simulink model "run_quadrotor_2020a"  (R2020a)
settings: Solver=ode23  StartTime=0.0  StopTime=60  FixedStep=10/1000  MaxStep=0.01  MinStep=1/1000  RelTol=1e-5  EnableMultiTasking=on
InitFcn:
  | addpath('display/')
  | addpath('parameters/')
  | addpath('quadrotor_model')
  | addpath('tools/')
  | addpath('libs/RealTima_Pacer')
  | aerosonde_parameters
  | simulation_parameters
model workspace (MAT data in the model file):
  D1_podbor1 = 902.0676
  D1_podbor_psi = 334.133298018
  D1_podbor_y = 97.9069
  D_podbor_x = 10
  D_podbor_z = 10
  I1_podbor1 = 320.9285
  I1_podbor_psi = 2.71828630961
  I1_podbor_y = 0.6752
  I_podbor_x = 50
  I_podbor_z = 50
  P1_podbor1 = 7509.4
  P1_podbor_psi = 848.547345881
  P1_podbor_y = 264.9363
  P_podbor_x = 50
  P_podbor_z = 50
  theta_1_P_param : Simulink.Parameter (value not decoded)
  theta_1_P_paramCopy : Simulink.Parameter (value not decoded)
undefined symbols (not defined in the file or in its folder): drawQuadrotor, filter_freq, ln, MAV, plotmavstatevariables, setup_pid
libraries: simulink x11, checkpacklib x5, dspsigattribs x2, realtime_pacer_lib x1
(part 2 of 2)

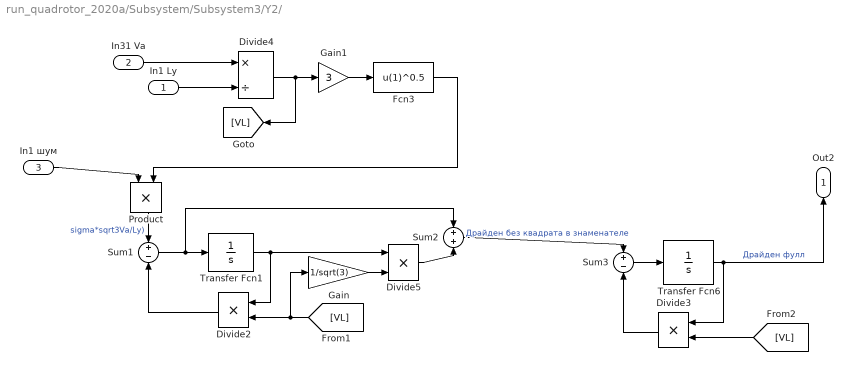
== system run_quadrotor_2020a/Subsystem/Subsystem3/Y2/  ==
  In1 Ly : Inport
  In31 Va : Inport  Port=2
  "In1 шум " : Inport  Port=3
  Divide2 : Product  Inputs=**
  Divide3 : Product  Inputs=**
  Divide4 : Product  Inputs=*/
  Divide5 : Product  Inputs=**
  Fcn3 : Fcn  Expr=u(1)^0.5
  Gain : Gain  Gain=1/sqrt(3)
  Gain1 : Gain  Gain=3
  Product : Product
  Sum1 : Sum  Inputs=+-
  Sum2 : Sum
  Sum3 : Sum  Inputs=+-
  Transfer Fcn1 : TransferFcn  Denominator="[1  0]"
  Transfer Fcn6 : TransferFcn  Denominator="[1  0]"
  Out2 : Outport
  wires:
  Divide4/1 -> [VL], Gain1/1
  Sum1/1 -> Transfer Fcn1/1, Sum2/1
  Sum2/1 -> Sum3/1  "Драйден без квадрата в знаменателе"
  Transfer Fcn1/1 -> Divide2/1, Divide5/1
  Divide2/1 -> Sum1/2
  Gain1/1 -> Fcn3/1
  In31 Va/1 -> Divide4/1
  In1 Ly/1 -> Divide4/2
  [VL] -> Gain/1, Divide2/2
  Gain/1 -> Divide5/2
  Divide5/1 -> Sum2/2
  Transfer Fcn6/1 -> Out2/1, Divide3/1  "Драйден фулл"
  Divide3/1 -> Sum3/2
  Sum3/1 -> Transfer Fcn6/1
  [VL] -> Divide3/2
  "In1 шум "/1 -> Product/1
  Fcn3/1 -> Product/2
  Product/1 -> Sum1/1  "sigma*sqrt3Va/Ly)"

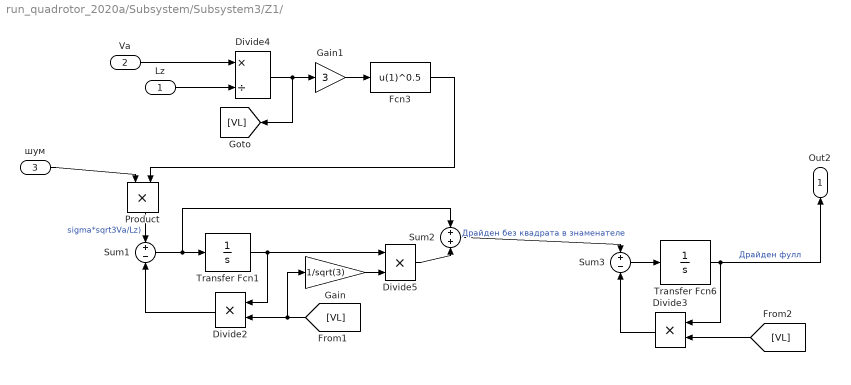
== system run_quadrotor_2020a/Subsystem/Subsystem3/Z1/  ==
  Lz : Inport
  Va : Inport  Port=2
  "шум " : Inport  Port=3
  Divide2 : Product  Inputs=**
  Divide3 : Product  Inputs=**
  Divide4 : Product  Inputs=*/
  Divide5 : Product  Inputs=**
  Fcn3 : Fcn  Expr=u(1)^0.5
  Gain : Gain  Gain=1/sqrt(3)
  Gain1 : Gain  Gain=3
  Product : Product
  Sum1 : Sum  Inputs=+-
  Sum2 : Sum
  Sum3 : Sum  Inputs=+-
  Transfer Fcn1 : TransferFcn  Denominator="[1  0]"
  Transfer Fcn6 : TransferFcn  Denominator="[1  0]"
  Out2 : Outport
  wires:
  Divide4/1 -> [VL], Gain1/1
  Sum1/1 -> Transfer Fcn1/1, Sum2/1
  Sum2/1 -> Sum3/1  "Драйден без квадрата в знаменателе"
  Transfer Fcn1/1 -> Divide2/1, Divide5/1
  Divide2/1 -> Sum1/2
  Gain1/1 -> Fcn3/1
  Va/1 -> Divide4/1
  Lz/1 -> Divide4/2
  [VL] -> Gain/1, Divide2/2
  Gain/1 -> Divide5/2
  Divide5/1 -> Sum2/2
  Transfer Fcn6/1 -> Out2/1, Divide3/1  "Драйден фулл"
  Divide3/1 -> Sum3/2
  Sum3/1 -> Transfer Fcn6/1
  [VL] -> Divide3/2
  "шум "/1 -> Product/1
  Fcn3/1 -> Product/2
  Product/1 -> Sum1/1  "sigma*sqrt3Va/Lz)"

== matlab function run_quadrotor_2020a/Subsystem1/In what the force, bro? ==
  data: Vb input; Fb output; Wb input
function Fb = AerialDrag(Vb, Wb)
    rho = 1.19;
    Va_vec = Vb - Wb;  % w - wind, v - ground speed; body frame
    Va = norm(Va_vec);
    alpha = atan2(Va_vec(2), Va_vec(1));    % attack angle
    beta = atan2(Va_vec(3), Va_vec(1));     % скольжения angle
    
    Va_0 = 10; % скорость, для которой рассчитаны зависимости сил
    rho_0 = 1.225;  % плотность воздуха при выведении зависимостей сил
%     C_0 = 0.715 / (0.5*rho_0*Va_0^2);  % if alpha = 0, beta = 0;
    % ----------------------------------------------------
    % alpha angle
    alpha = abs(alpha);
    alpha = sign(alpha)*mod(alpha, 180);
    alpha = alpha + 180 * sign(90-alpha)*(abs(alpha)>90);
    if alpha >= 0 && alpha <= 20
        F_xy = 0.6969 + 0.0022*(alpha+2.3409).^2;
    elseif alpha > 20 && alpha <= 90
        F_xy = -0.000435*alpha^2 + 0.098161*alpha - 0.007685;
%         C_d = 5.5300 - 4.3500e-04*(alpha - 112.8287)^2;
    elseif alpha >= -20 && alpha < 0
        F_xy = 0.6969 + 0.0022*(-alpha+2.3409).^2;
    else
        F_xy = 5.5300 - 4.3500e-04*(-alpha - 112.8287)^2;
    end
%     C_D_alpha = F_0 / (0.5*rho_0*Va_0^2) - C_0;
%     C_D_alpha = F_0 / (0.5*rho_0*Va_0^2);
        C_xy = F_xy / (0.5*rho_0*Va_0^2);
        C_x = C_xy * cos(alpha);
        C_y = C_xy * sin(alpha);
        
        
    
    %-----------------------------------------------------
    % beta angle
    b = abs(beta);
    b = sign(b)*mod(b, 180);
    b = b + 180 * sign(90-b)*(abs(b)>90);
    if b >= 0 && b <= 10
        F_xz = 2.81659e-7*b^6 - 5.42002e-6*b^5 + 0.0000194033*b^4 + 0.000149284*b^3 - 0.000766659*b^2 + 0.00100311*b + 0.715;
    elseif b > 10 && b <= 32
        F_xz = 0.000072941364*b^2+0.004725990899*b+0.676768850038;
    elseif b > 32 && b <= 47
        F_xz = 0.000014983590*b^3-0.002016505717*b^2+0.091338487517*b-0.446303186240;
    elseif b > 47 && b <= 66
        F_xz = -0.000005286789*b^3+0.000705178007*b^2-0.030877630605*b+1.390205322532;
    elseif b > 66 && b <= 90
        F_xz = 0.000000379469*b^3+0.000021666922*b^2-0.013615025702*b+1.599215019960;            
    else
        F_xz = 0;
    end
    C_xz = F_xz / (0.5*rho_0*Va_0^2);
    C_z = C_xz * sin(beta);
%     C_D_beta = F0 / (0.5*rho_0*Va_0^2) - C_0;
    
    
    % ----------------------------------------------
    % Drug force
%     F_D = 0.5*rho*Va^2 * (C_0 + alpha*C_D_alpha + beta*C_D_beta);
    
%     F_D = 0.5*rho*Va^2 * (C_D_alpha);
%     
%     Fa = [
%         (-1)*F_D;
%         0;
%         0;
%     ];  % в скоростной СК
%     c_a = cos(alpha); s_a = sin(alpha);
%     c_b = cos(beta); s_b = sin(beta);
%     % TODO: перепроверить, кто в кого переводитъ
%     R_a_b = [c_a*c_b -s_a*c_b s_b; s_a c_a 0; -c_a*s_b s_a*s_b c_b];    % из скоростной с связанную
% %     R_b_a = [ c_a s_a 0; -s_a c_a 0; 0 0 1];    % из связанной в скоростную
% %     Fb = R_b_a' * Fa;
%         Fb = R_a_b * Fa;
    Fb = (-1)*(1/2)*rho*Va^2 * [C_x; C_y; C_z];
end

== matlab function run_quadrotor_2020a/Motor Controller1 ==
  data: N output; u input
% Calculate desired motor speeds N with given control u
function N = fcn(u)
u_T = u(1);
u_x = u(2);
u_y = u(3);
u_z = u(4);

% NN = 0.25*[u_T+u_z u_T+u_z u_T-u_z u_T-u_z]';
% A = (1/4)*[
%     1 1;
%     1 1;
%     1 -1;
%     1 -1
% ];
A = (1/4)*[
    1 1 1 1;
    1 -1 -1 1;
    1 -1 1 -1;
    1 1 -1 -1;
];

NN = A*[u_T; u_x; u_y; u_z];
NN = max(NN, 0);
N = sqrt(NN);

% If we want at once disarm motors (landing etc.)
% if disable_motors == 7
%     N = zeros(4,1);
% end

== matlab function run_quadrotor_2020a/REG1/Flush integrators commandor/MATLAB Function ==
  data: mode_vec input; prev_mode_vec input; command output; prev_command input; mode_vec output
function [command, mode_vec]  = fcn(mode_vec, prev_mode_vec, prev_command)
    command = prev_command;
%     persistent prev_mode;
%     if isempty(prev_mode)
%        prev_mode = -1; 
%     end
    if prev_mode_vec == mode_vec
        return
    end
%     prev_mode = mode;
    % command: [ theta x y]
    
    mode = FlightMode(mode_vec);
    prev_mode = FlightMode(prev_mode_vec);
    phi = 1; x = 2; y = 3;
    
    % если изменился канал х
    if mode.get('x') ~= prev_mode.get('x')
        command(x) = double(~prev_command(x));
        if mode.get('x') == 0 || mode.get('x') == 1
            command(phi) = double(~prev_command(phi));
        end
    end
    
    if mode.get('y') ~= prev_mode.get('y')
        command(y) = double(~prev_command(y));
    end
    
    

%     if mode == 2 || mode == 0
%         command = double(~prev_command);
%     end
%     if mode == 3 || mode == 5
%         command(2) = double(~prev_command(2));
%     end
%     if mode == 4 || mode == 5 || mode == 6
%         command(3) = double(~prev_command(3));
%     end

== matlab function run_quadrotor_2020a/Subsystem/Subsystem3/MATLAB Function1 ==
  data: euler input; Wb output; va input
function Wb = rotate_g_b(euler, va)
R = getRotationMatrix(euler);
vay=0; vaz=0;
Va = [-va; vay; vaz];
Wb = R*Va;

function R = getRotationMatrix(angles)
    phi = 1; t = 2; psi = 3; %indices
    s = sin(angles);
    c = cos(angles);
    R = [
        c(t)*c(psi) s(t)    -c(t)*s(psi);
        -c(phi)*s(t)*c(psi)+s(phi)*s(psi) c(phi)*c(t) c(phi)*s(t)*s(psi)+s(phi)*c(psi);
        s(phi)*s(t)*c(psi)+c(phi)*s(psi)  -s(phi)*c(t)    -s(psi)*s(t)*s(phi)+c(psi)*c(phi);
    ];

== matlab function run_quadrotor_2020a/Subsystem1/Old Force ==
  data: v input; F output; w input
function F = AerialDrag(v, w)
    rho = 1.19;
    S = [5573 59852 6884] / (100*10)^2;
    C = 1.0;
    Va = v - w;  % w - wind, v - ground speed;
    % S - характерная площадь
    F = - C * rho * Va.^2/2 .* S';
end

== matlab function run_quadrotor_2020a/REG1/g -> g_1(psi) ==
  data: g_vec input; g1_vec output; psi input
% Поворот вектора глобальной СК в полусвязанную на угол рыскания
function g1_vec = fcn(g_vec, psi)

c_p = cos(psi); s_p = sin(psi);
R = [c_p 0 -s_p; 0 1 0; s_p 0 c_p];
g1_vec = R * g_vec;

== matlab function run_quadrotor_2020a/Sensors Real/MATLAB Function ==
  data: v input; d_v input; ang input; a_prop output; w input
% Считает проекции кажущегося ускорения,
% эмуляция показателей акселерометра
% @v - скорость в связанной СК
% @d_v - производная скорости выше
% @ang - углы Эйлера
% @w - угловая скорость в проекциях на связанные оси
function a_prop = fcn(v, d_v, ang, w)
phi = ang(1);
theta = ang(2); 
g = 9.81;

% coriolis = [
%     w(3)*v(2) - w(2)*v(3);
%     w(1)*v(3) - w(3)*v(1);
%     w(2)*v(1) - w(1)*v(2)
% ];

coriolis = cross(v, w);

R = [
    sin(theta);
    cos(phi)*cos(theta);
    -sin(phi)*cos(theta)
];

a_prop = d_v - coriolis + R*g;

% a_prop(1) = d_v(1) - (w(3)*v(2) - w(2)*v(3)) + g*sin(theta);
% a_prop(2) = d_v(2) - (w(1)*v(3) - w(3)*v(1)) + g*cos(phi)*cos(theta);
% a_prop(3) = d_v(3) - (w(2)*v(1) - w(1)*v(2)) - g*sin(phi)*cos(theta);

== matlab function run_quadrotor_2020a/desired fixed1 ==
  data: des_state output; MAV parameter
function des_state = fcn(  MAV)

% pos = [8  0 5.87]';
pos = [MAV.x0+0.2  MAV.y0 MAV.z0+0.2]';
vel = [0 0 0]';
acc = [0 0 0]';
des_state = [pos vel acc];

== matlab function run_quadrotor_2020a/Target/Target equations ==
  data: t input; t0 input; r output; r0 input; v0 input; a0 input; dr output; ddr output
 function [ r, dr, ddr] = fcn(t, t0, r0, v0, a0)
    t = max(0, t - t0);
    r = r0 + v0*t + a0*t.^2/2;
    dr = v0 + a0*t;
    ddr = [0 0 0]';

== matlab function run_quadrotor_2020a/REG1/MATLAB Function ==
  data: psi input; phi_c output; xi input; xi_dot input; Vg input
function phi_c = fcn(psi, xi, xi_dot, Vg)

phi = atan(xi_dot * Vg / (9.81*cos(psi - xi)));
phi_c = [phi; 0];

== matlab function run_quadrotor_2020a/REG1/MATLAB Function1 ==
  data: x input; V output; y input; z input
function V = fcn(x, y, z)

V = sqrt(x.^2 + y.^2 + z.^2);

== matlab function run_quadrotor_2020a/REG1/MATLAB Function2 ==
  data: x_des input; psi_c output; z_des input; x input; z input
function psi_c = fcn(x_des, z_des, x, z)

psi_c = [atan2(-z_des+z, -x_des+x)];

== matlab function run_quadrotor_2020a/MATLAB Function ==
  data: state input; desired output; n input; n output
function [desired, n] = fcn(state, n)

x = state(1); y = state(2); z = state(3);
r = [x y z]';

% select r_desired_prev

r_des = get_square_traj(n);
if norm(r_des - r) < 0.4
    n = n + 1;
%     r_des = get_circle_traj(n);
    r_des  =get_square_traj(n);
end

desired = [r_des [0 0 0]' [0 0 0]'];

end

function r_des = get_circle_traj(n)
    R = 10;
    N = 100;
    r_des = [
        R*cos(2*pi/N*n);
        0;
        R*sin(2*pi/N*n)
    ];
end

function r_des = get_square_traj(n)
    a = 10;
    map = [
        a 0 0;
        a a a;
        0 a a;
        0 0 0;
        a 0 0;
    ]';
    r_des = map(:, n + 1);
end

== matlab function run_quadrotor_2020a/Quadrotor/MATLAB Function ==
  data: t input; x input; uu input; y output; MAV parameter
function y  = mdlDerivatives(t, x, uu, MAV)    
%   Earth coordinates
    pn    = x(1);
    pe    = x(2);
    pd    = x(3);
%   speed in 'b' coordinates
    u     = x(4);
    v     = x(5);
    w     = x(6);
%   position quaternions
    phi    = x(7);
    theta    = x(8);
    psi    = x(9);
%   angular speeds
    p     = x(10);  % крен
    q     = x(11);  % рыскание
    r     = x(12);  % тангаж

    N = uu(1:4);
    
    wind = uu(5:7);
    R_g_b = Utils.getRotationMatrix([phi theta psi]);   % матрица поворота (g->b) {из Земной нормальной в связанную СК}

    cache.R_g_b = R_g_b;
    [Fb, Mb] = forces_moments(t,x,uu, wind, MAV, cache);
    
    % поступательная кинематика
    p_dot = R_g_b' * [u v w]';
    
    pn_dot = p_dot(1); pe_dot = p_dot(2); pd_dot = p_dot(3);    % x y z
    
    % вращательная кинематика
    tmp_matrix = [
        1, -cos(phi)*tan(theta), sin(phi)*tan(theta);
        0, cos(phi)/cos(theta),  -sin(phi)/cos(theta);
        0, sin(phi),             cos(phi)
    ];
    euler_angles = tmp_matrix * [p q r]';
    phi_dot = euler_angles(1); 
    psi_dot = euler_angles(2); theta_dot =  euler_angles(3);
    
    % поступательная динамика
    speed_dot = hat([u v w]')*[p q r]' + (1/MAV.mass) * Fb;
    u_dot = speed_dot(1); v_dot = speed_dot(2); w_dot = speed_dot(3);
    
    % вращательная динамика
    pqr_dot = MAV.J_inv * ( hat([p q r]) * MAV.J * [p q r]' + Mb );
    p_dot = pqr_dot(1); q_dot = pqr_dot(2); r_dot = pqr_dot(3);

    y = [ ...
            pn_dot pe_dot pd_dot        ...
            u_dot v_dot w_dot           ...
            phi_dot theta_dot psi_dot   ...
            p_dot q_dot r_dot           ...
          ]';
end

% @return: Вектора силы и момента в связанной СК
function [Fb, Mb] = forces_moments(t,x,uu, wind_speed, MAV, cache)
    N = uu(1:4);    % скорость вращения двигов
    Omega = 2*pi*N/60;
    R_g_b = cache.R_g_b;
    
    % Forces
    f_gravity = R_g_b * [0; MAV.mass*(-MAV.gravity); 0];
    f = Gaurang(N, MAV.Prop, MAV.rho, x(5));
    f_thrust = [0 1 0]' * sum(f);
%     P_thrust = [0; 1; 0] * sum(f_thrust);   % тяго
%     wind = R_g_b * MAV.Env.Wind_speed;
    wind = wind_speed;
    f_aerial_drag = AerialDrag(x(4:6), wind, MAV.rho);
% f_aerial_drag = AerialDrag(x(4:6), wind, MAV.rho, MAV.Body.S, MAV.Body.C_aerial_drag_1);
    Fb = f_gravity + f_aerial_drag + f_thrust;    % результирующая сил в связанной СК

    % Moments
    
%     M_gyro = [mx my mz]';  % от винтов, вращение по рЫсканию
%     M_gyro = m;
    % отключено временно
%     M_y_aerial_vec = PropellerAeroMomentumPlain(N, MAV.Prop, MAV.rho); % за счет аэродинамического сопротивления
%     M_y_aerial = (-1) * sum(MAV.Prop.K_direction .*  M_y_aerial_vec);

    M_y_aerial = PropellerAeroMomentunParabole(N, MAV.Prop); % экспериментально подобранная зависимость, по факту включает в себя момент инерции
    
%     M_y_inertia = (MAV.Prop.J_y + MAV.Motor.J_rotor) .* sum(MAV.Prop.K_direction .* Omega.^2)
    M_y_inertia = 0;
%     M_y_aerial = 0;

    M_motors = [0 1 0]' * (M_y_aerial + M_y_inertia);

    M_gyro = [0 0 0]';

    M_traction = [
        ( f(1) + f(4) - (f(2) + f(3)) ) * MAV.radius_z*1e-3;
        0;
        ( f(1) + f(2) - (f(3) + f(4)) ) * MAV.radius_x*1e-3;
    ];

    

    Mb = M_gyro + M_traction + M_motors;
end

% Вычисление силы тяги по методу Gaurang
function T = Gaurang(N, prop, rho, Va)
    persistent K_f
    if isempty(K_f)
        d = prop.d;
        p = prop.p;
        ed = prop.ed;
        k = prop.Nb * prop.c_d / 2;
        theta = atan(p/(pi*d));
        %     lambda_c = Va./(Omega*d/2);
        lambda_c = 0;

        C_T = 4/3*k*theta*(1 - (1 - ed)^3) - ...
              k*( sqrt((lambda_c + k).^2+k) - sqrt(k) ) * (1-(1-ed)^2);

        K_f = 1/6*rho*pi*(ed*d/2)^4*C_T;
        K_f = K_f * prop.K;
    end

    Omega = 2*pi*N/60;
    T = Omega.^2 .* K_f;
end

function M = PropellerAeroMomentunParabole(N, Prop)
%     Omega = 2*pi*N/60;
    M = [1 -1 1 -1] * (Prop.C_aerial_momentum*(N + Prop.A_drift).^2);
end

function M = PropellerAeroMomentumPlain(N, prop, rho)
    C = prop.C_1;
    S = prop.S_approx * sin(atan(prop.p/(pi*prop.d)));
    Omega = 2*pi*N/60;

    F = 1/2 * rho * S * C * (prop.d/2*Omega).^2;
    m_p = 3/4;      % точка приложения момента воздухом к винту
    M = F * (prop.d/2 * m_p);
end

% Сила аэродинамического сопротивления
% function F = AerialDrag(v, w, rho, S, C)
%     Va = v - w;  % w - wind, v - ground speed;
%     % S - характерная площадь
%     F = - C * rho * Va.^2/2 .* S';
%     
% end
function Fb = AerialDrag(Vb, Wb, rho)
    Va_vec = Vb - Wb;  % w - wind, v - ground speed; body frame
    Va = norm(Va_vec);
    alpha = atan2(Va_vec(2), Va_vec(1));    % attack angle
    % alpha angle
    if alpha >= 0 && alpha <= 20
        F_0 = 0.6969 + 0.0022*(alpha+2.3409).^2;
    elseif alpha >= -45 && alpha < 0
        F_0 = 0.6969 + 0.0022*(-alpha+2.3409).^2;
    elseif alpha > 20 && alpha <= 90
        F_0 = -0.000435*alpha^2 + 0.098161*alpha - 0.007685;
%         C_d = 5.5300 - 4.3500e-04*(alpha - 112.8287)^2;
    else
        F_0 = 5.5300 - 4.3500e-04*(-alpha - 112.8287)^2;
    end
    C_D_alpha = F_0 / (0.5*rho*Va^2);
    F_D = 0.5*rho*C_D_alpha*Va^2;
    
    Fa = [
        (-1)*F_D;
        0;
        0;
    ];  % в скоростной СК
    c_a = cos(alpha); s_a = sin(alpha);
    R_b_a = [ c_a s_a 0; -s_a c_a 0; 0 0 1];    % из связанной в скоростную
    Fb = R_b_a' * Fa;
    Fb = Fb*2;
    
end
